simulink model "Cinematica"  (R2020b)
settings: Solver=VariableStepAuto  StartTime=0.0  StopTime=Smi.general.simulation_time  FixedStep=0.001  MaxStep=0.001  RelTol=1e-3  AbsTol=1e-3  EnableMultiTasking=on
undefined symbols (not defined in the file or in its folder): Smi, X, Y, Z
libraries: sm_lib x99, nesl_utility x24, simulink x1, dspsrcs4 x1, cstblocks x1
(part 5 of 5)

== system Cinematica/FIXED CHASSIS/BODY/FL HARDPOINTS/C forces sensing ==
  F : Inport
  Demux : Demux  Outputs=3
  To Workspace : ToWorkspace  VariableName=FL_C_Fx  SaveFormat=Timeseries  SampleTime=-1
  To Workspace1 : ToWorkspace  VariableName=FL_C_Fy  SaveFormat=Timeseries  SampleTime=-1
  To Workspace2 : ToWorkspace  VariableName=FL_C_Fz  SaveFormat=Timeseries  SampleTime=-1
  wires:
  Demux/1 -> To Workspace/1
  Demux/3 -> To Workspace2/1
  Demux/2 -> To Workspace1/1
  F/1 -> Demux/1

== system Cinematica/FIXED CHASSIS/BODY/FL HARDPOINTS/D forces sensing ==
  F : Inport
  Demux : Demux  Outputs=3
  To Workspace : ToWorkspace  VariableName=FL_D_Fx  SaveFormat=Timeseries  SampleTime=-1
  To Workspace1 : ToWorkspace  VariableName=FL_D_Fy  SaveFormat=Timeseries  SampleTime=-1
  To Workspace2 : ToWorkspace  VariableName=FL_D_Fz  SaveFormat=Timeseries  SampleTime=-1
  wires:
  Demux/1 -> To Workspace/1
  Demux/3 -> To Workspace2/1
  Demux/2 -> To Workspace1/1
  F/1 -> Demux/1

== system Cinematica/FIXED CHASSIS/BODY/FL HARDPOINTS/crank forces sensing ==
  F : Inport
  Demux : Demux  Outputs=3
  To Workspace : ToWorkspace  VariableName=FL_CRANK_Fx  SaveFormat=Timeseries  SampleTime=-1
  To Workspace1 : ToWorkspace  VariableName=FL_CRANK_Fy  SaveFormat=Timeseries  SampleTime=-1
  To Workspace2 : ToWorkspace  VariableName=FL_CRANK_Fz  SaveFormat=Timeseries  SampleTime=-1
  wires:
  Demux/1 -> To Workspace/1
  Demux/3 -> To Workspace2/1
  Demux/2 -> To Workspace1/1
  F/1 -> Demux/1

== system Cinematica/FIXED CHASSIS/BODY/FL HARDPOINTS/damper forces sensing ==
  F : Inport
  Demux : Demux  Outputs=3
  To Workspace : ToWorkspace  VariableName=FL_AMMO_Fx  SaveFormat=Timeseries  SampleTime=-1
  To Workspace1 : ToWorkspace  VariableName=FL_AMMO_Fy  SaveFormat=Timeseries  SampleTime=-1
  To Workspace2 : ToWorkspace  VariableName=FL_AMMO_Fz  SaveFormat=Timeseries  SampleTime=-1
  wires:
  Demux/1 -> To Workspace/1
  Demux/3 -> To Workspace2/1
  Demux/2 -> To Workspace1/1
  F/1 -> Demux/1
